simulink model "Team23_project2_final"  (R2023b)
settings: Solver=VariableStepAuto  StartTime=0.0  StopTime=10.0  RelTol=1e-3
undefined symbols (not defined in the file or in its folder): carData
settings Model: Creator=vince  LastModifiedBy=kkern

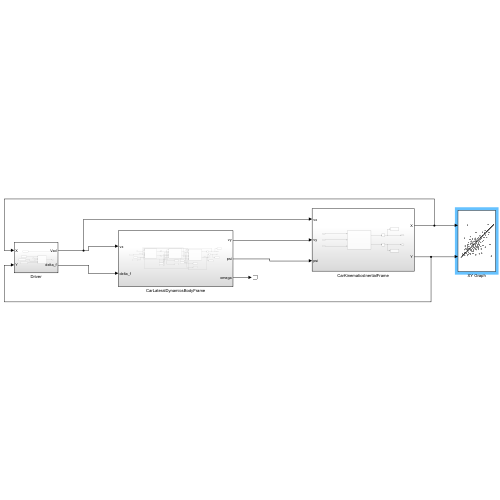
[thumbnail: Simulink's stored preview of the top-level diagram]
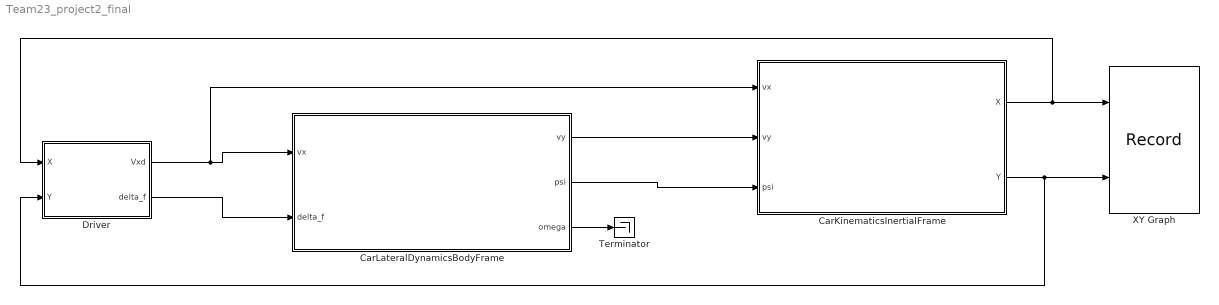
== system Team23_project2_final ==
  CarKinematicsInertialFrame : Subsystem
  CarLateralDynamicsBodyFrame : Subsystem
  Driver : Subsystem
  Terminator : Terminator
  XY Graph : Record  FileSettingsInternal="{\"entries\":[{\"content\":{\"excelSettings\":{\"content\":{},\"type\":\"Streamout.ExcelSettings\"}},\"type\":\"Streamout.FileSettingStorage\",\"uuid\":\"\"}],\"packageUris\":[\"http:\\/\\/schema.mathworks.com\\/mf0\\/streamout_blocks\\/R2020a\"],\"version\":\"1.0\"}"  Layout=[1 1]  SignalsInternal="{\"entries\":[{\"content\":{\"signals\":[{\"content\":{\"blockPath\":[],\"dimensions\":[1],\"domain\":\"\",\"lineColor\":\"#a2142f\",\"port\":1,\"sid\":[\"\"],\"signalID\":251,\"signalName\":\"CarKinematicsInertialFrame:1\"},\"type\":\"RecordBlkView.Signal\",\"uuid\":\"\"},{\"content\":{\"blockPath\":[],\"dimensions\":[1],\"domain\":\"\",\"lineColor\":\"#139fff\",\"port\":2,\"sid\":[\"\"],\"signalID\":255,\"signalName\":\"CarKinematicsInertialFrame:2\"},\"type\":\"RecordBlkView.Signal\",\"uuid\":\"\"}]},\"type\":\"RecordBlkView.InputSignals\",\"uuid\":\"\"}],\"packageUris\":[\"http:\\/\\/schema.mathworks.com\\/mf0\\/streamout_blocks\\/R2020a\"],\"version\":\"1.0\"}"  VisualizationBindings="{\"xyplotplugin\":{\"info\":[{\"series\":[],\"subplotID\":1}]}}"  CompatibilityTag=XY
  wires:
  CarKinematicsInertialFrame/1(X) -> Driver/1(X), XY Graph/1
  CarKinematicsInertialFrame/2(Y) -> Driver/2(Y), XY Graph/2
  CarLateralDynamicsBodyFrame/2(psi) -> CarKinematicsInertialFrame/3(psi)
  CarLateralDynamicsBodyFrame/1(vy) -> CarKinematicsInertialFrame/2(vy)
  CarLateralDynamicsBodyFrame/3(omega) -> Terminator/1
  Driver/2(delta_f) -> CarLateralDynamicsBodyFrame/2(delta_f)
  Driver/1(Vxd) -> CarKinematicsInertialFrame/1(vx), CarLateralDynamicsBodyFrame/1(vx)

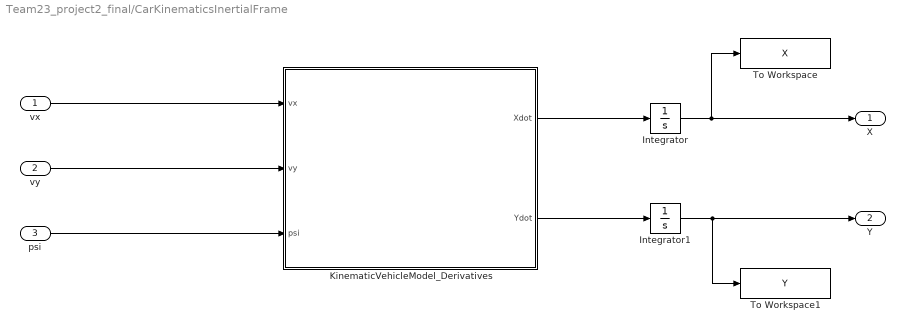
== system Team23_project2_final/CarKinematicsInertialFrame ==
  vx : Inport
  vy : Inport  Port=2
  psi : Inport  Port=3
  Integrator : Integrator
  Integrator1 : Integrator
  KinematicVehicleModel_Derivatives : MATLAB Function  TreatAsAtomicUnit=on
  To Workspace : ToWorkspace  VariableName=X  SaveFormat=Timeseries  SampleTime=-1
  To Workspace1 : ToWorkspace  VariableName=Y  SaveFormat=Timeseries  SampleTime=-1
  X : Outport
  Y : Outport  Port=2
  wires:
  vx/1 -> KinematicVehicleModel_Derivatives/1(vx)
  vy/1 -> KinematicVehicleModel_Derivatives/2(vy)
  psi/1 -> KinematicVehicleModel_Derivatives/3(psi)
  KinematicVehicleModel_Derivatives/1(Xdot) -> Integrator/1
  KinematicVehicleModel_Derivatives/2(Ydot) -> Integrator1/1
  Integrator/1 -> To Workspace/1, X/1
  Integrator1/1 -> To Workspace1/1, Y/1

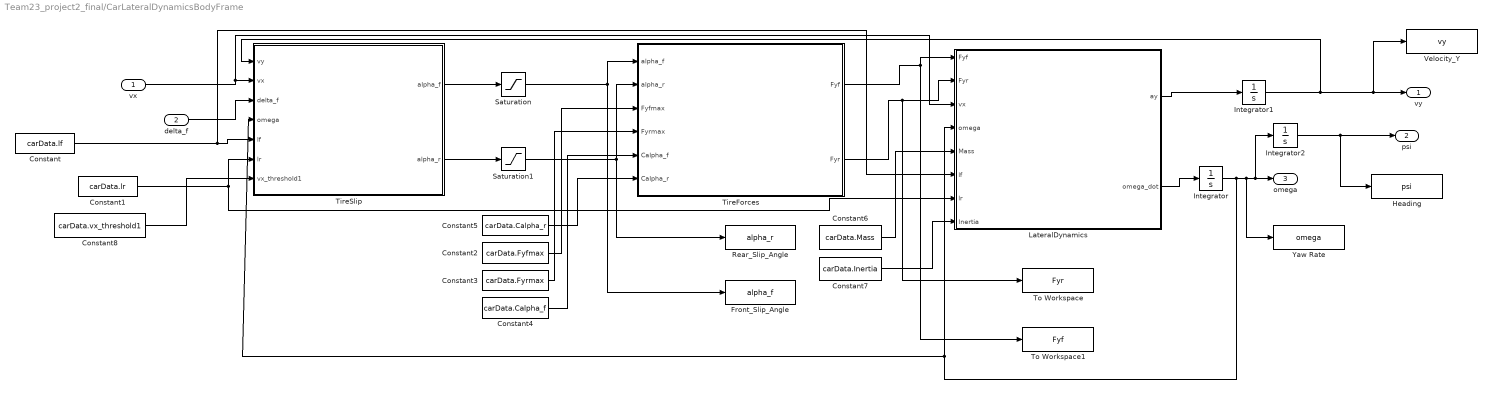
== system Team23_project2_final/CarLateralDynamicsBodyFrame ==
  vx : Inport
  delta_f : Inport  Port=2
  Constant : Constant  Value=carData.lf
  Constant1 : Constant  Value=carData.lr
  Constant2 : Constant  Value=carData.Fyfmax
  Constant3 : Constant  Value=carData.Fyrmax
  Constant4 : Constant  Value=carData.Calpha_f
  Constant5 : Constant  Value=carData.Calpha_r
  Constant6 : Constant  Value=carData.Mass
  Constant7 : Constant  Value=carData.Inertia
  Constant8 : Constant  Value=carData.vx_threshold1
  Front_Slip_Angle : ToWorkspace  VariableName=alpha_f  SaveFormat=Timeseries  SampleTime=-1
  Heading : ToWorkspace  VariableName=psi  SaveFormat=Timeseries  SampleTime=-1
  Integrator : Integrator
  Integrator1 : Integrator
  Integrator2 : Integrator
  LateralDynamics : MATLAB Function  TreatAsAtomicUnit=on
  Rear_Slip_Angle : ToWorkspace  VariableName=alpha_r  SaveFormat=Timeseries  SampleTime=-1
  Saturation : Saturate  UpperLimit=0.0698  LowerLimit=-0.0698
  Saturation1 : Saturate  UpperLimit=0.0698  LowerLimit=-0.0698
  TireForces : MATLAB Function  TreatAsAtomicUnit=on
  TireSlip : MATLAB Function  TreatAsAtomicUnit=on
  To Workspace : ToWorkspace  VariableName=Fyr  SaveFormat=Timeseries  SampleTime=-1
  To Workspace1 : ToWorkspace  VariableName=Fyf  SaveFormat=Timeseries  SampleTime=-1
  Velocity_Y : ToWorkspace  VariableName=vy  SaveFormat=Timeseries  SampleTime=-1
  Yaw Rate : ToWorkspace  VariableName=omega  SaveFormat=Timeseries  SampleTime=-1
  vy : Outport
  psi : Outport  Port=2
  omega : Outport  Port=3
  wires:
  delta_f/1 -> TireSlip/3(delta_f)
  TireSlip/2(alpha_r) -> Saturation1/1
  TireForces/1(Fyf) -> LateralDynamics/1(Fyf), To Workspace1/1
  TireForces/2(Fyr) -> LateralDynamics/2(Fyr), To Workspace/1
  vx/1 -> TireSlip/2(vx), LateralDynamics/3(vx)
  LateralDynamics/1(ay) -> Integrator1/1
  LateralDynamics/2(omega_dot) -> Integrator/1
  Integrator2/1 -> Heading/1, psi/1
  Integrator1/1 -> TireSlip/1(vy), Velocity_Y/1, vy/1
  Integrator/1 -> LateralDynamics/4(omega), TireSlip/4(omega), Yaw Rate/1, Integrator2/1, omega/1
  TireSlip/1(alpha_f) -> Saturation/1
  Constant1/1 -> TireSlip/6(lr), LateralDynamics/7(lr)
  Constant/1 -> TireSlip/5(lf), LateralDynamics/6(lf)
  Constant5/1 -> TireForces/6(Calpha_r)
  Constant2/1 -> TireForces/3(Fyfmax)
  Constant3/1 -> TireForces/4(Fyrmax)
  Constant4/1 -> TireForces/5(Calpha_f)
  Constant7/1 -> LateralDynamics/8(Inertia)
  Constant6/1 -> LateralDynamics/5(Mass)
  Saturation/1 -> TireForces/1(alpha_f), Front_Slip_Angle/1
  Saturation1/1 -> TireForces/2(alpha_r), Rear_Slip_Angle/1
  Constant8/1 -> TireSlip/7(vx_threshold1)

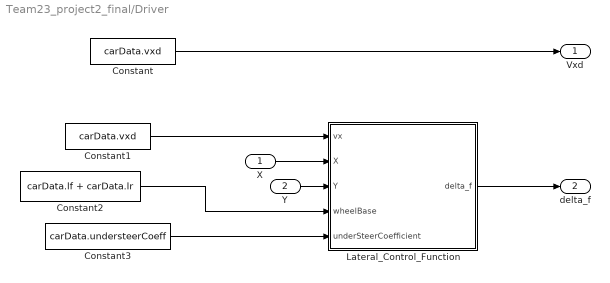
== system Team23_project2_final/Driver ==
  X : Inport
  Y : Inport  Port=2
  " Lateral_Control_Function" : MATLAB Function  TreatAsAtomicUnit=on
  Constant : Constant  Value=carData.vxd
  Constant1 : Constant  Value=carData.vxd
  Constant2 : Constant  Value=carData.lf + carData.lr
  Constant3 : Constant  Value=carData.understeerCoeff
  Vxd : Outport
  delta_f : Outport  Port=2
  wires:
  Constant1/1 -> " Lateral_Control_Function"/1(vx)
  Constant2/1 -> " Lateral_Control_Function"/4(wheelBase)
  Constant3/1 -> " Lateral_Control_Function"/5(underSteerCoefficient)
  " Lateral_Control_Function"/1(delta_f) -> delta_f/1
  X/1 -> " Lateral_Control_Function"/2(X)
  Y/1 -> " Lateral_Control_Function"/3(Y)
  Constant/1 -> Vxd/1

== matlab function Team23_project2_final/CarKinematicsInertialFrame/KinematicVehicleModel_Derivatives ==
  data: vx input; Xdot output; vy input; psi input; Ydot output
function [Xdot, Ydot] = fcn(vx, vy, psi)
    temp = TF(psi) * [vx;vy];
    Xdot = temp(1);
    Ydot = temp(2);
end

function y = TF(psi)
    y = [cos(psi), -sin(psi); sin(psi), cos(psi)];
end

== matlab function Team23_project2_final/CarLateralDynamicsBodyFrame/TireSlip ==
  data: vy input; alpha_f output; vx input; delta_f input; omega input; lf input; alpha_r output; lr input; vx_threshold1 input
function [alpha_f, alpha_r] = fnc(vy, vx, delta_f, omega, lf, lr, vx_threshold1)

    if abs(vx) > vx_threshold1
        alpha_f = delta_f - (vy + omega * lf) / vx;
        alpha_r = - (vy - omega * lr) / vx;
    else
        alpha_f = 0;
        alpha_r = 0;
    end

end

== matlab function Team23_project2_final/CarLateralDynamicsBodyFrame/TireForces ==
  data: alpha_f input; Fyf output; alpha_r input; Fyfmax input; Fyr output; Fyrmax input; Calpha_f input; Calpha_r input
function [Fyf, Fyr] = fcn(alpha_f, alpha_r, Fyfmax, Fyrmax, Calpha_f, Calpha_r)

    Fyf = min(Fyfmax, Calpha_f * alpha_f);
    Fyr = min(Fyrmax, Calpha_r * alpha_r);

end

== matlab function Team23_project2_final/CarLateralDynamicsBodyFrame/LateralDynamics ==
  data: Fyf input; ay output; Fyr input; vx input; omega input; Mass input; omega_dot output; lf input; lr input; Inertia input
function [ay, omega_dot] = fcn(Fyf, Fyr, vx, omega, Mass, lf, lr, Inertia)

    Fy = Fyf + Fyr;
    ay = Fy / Mass - omega * vx;

    M = Fyf * lf - Fyr * lr;
    omega_dot = M / Inertia;

end

== matlab function Team23_project2_final/Driver/ Lateral_Control_Function ==
  data: vx input; X input; delta_f output; Y input; wheelBase input; underSteerCoefficient input
function delta_f = latControl(vx, X, Y, wheelBase, underSteerCoefficient)

track_radius = 200;
track_length = 900;

track_seg1_x0 = 0;
track_seg1_y0 = 0;
track_seg1_x1 = track_length;
track_seg1_y1 = 0;
track_seg2_x0 = track_seg1_x1;
track_seg2_y0 = track_seg1_y1;
track_seg2_x1 = track_seg2_x0;
track_seg2_y1 = track_seg2_y0 + 2 * track_radius;
track_seg3_x0 = track_seg2_x1;
track_seg3_y0 = track_seg2_y1;
track_seg3_x1 = track_seg3_x0 - track_length;
track_seg3_y1 = track_seg3_y0;
track_seg4_x0 = track_seg3_x1;
track_seg4_y0 = track_seg3_y1;
track_seg4_x1 = track_seg1_x0;
track_seg4_y1 = track_seg1_y0;

if X > track_seg1_x0
    if X > track_seg1_x1
        segment = 2;
    else 
        if Y > (track_seg2_y0 + track_seg2_y1)/2
            segment = 3;
        else 
            segment = 1;
        end
    end
else
    segment = 4;
end


switch(segment)
    case 1
        delta_f = 0;
    case 2
        delta_f = - (wheelBase / track_radius + 1 * underSteerCoefficient * vx^2);
    case 3
        delta_f = 0;
    case 4
        delta_f = - (wheelBase / track_radius + 1 * underSteerCoefficient * vx^2);
    otherwise
        delta_f = 0;
end
